simulink model "differential_drive_base_robot_current_loop"  (R2015b)
settings: Solver=VariableStepAuto  StartTime=0.0  StopTime=10.0  RelTol=1e-3
values from neighbouring files (symbols this model uses):
  B = 0.1    [andbot1dot2_modeling_param.m]    (also in andbot1dot2_param.m)
  J = 0.1    [andbot1dot2_modeling_param.m]    (also in andbot1dot2_param.m)
  m = 18.8    [andbot1dot2_modeling_param.m]    (also in andbot1dot2_param.m)
  r = 0.085    [andbot1dot2_modeling_param.m]    (also in andbot1dot2_param.m)
undefined symbols (not defined in the file or in its folder): km
settings Model: Creator=shangwei  LastModifiedBy=shangwei

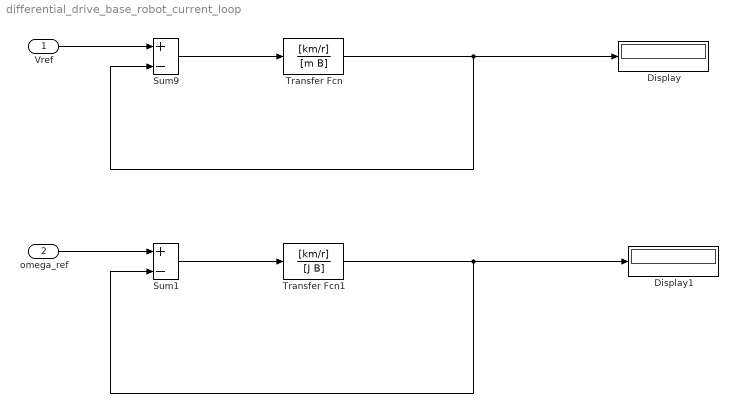
== system differential_drive_base_robot_current_loop ==
  Vref : Inport
  omega_ref : Inport  Port=2
  Display : Display
  Display1 : Display
  Sum1 : Sum  Inputs=+-
  Sum9 : Sum  Inputs=+-
  Transfer Fcn : TransferFcn  Numerator=[km/r]  Denominator=[m B]
  Transfer Fcn1 : TransferFcn  Numerator=[km/r]  Denominator=[J B]
  wires:
  Sum9/1 -> Transfer Fcn/1
  Transfer Fcn/1 -> Sum9/2, Display/1
  Vref/1 -> Sum9/1
  Sum1/1 -> Transfer Fcn1/1
  omega_ref/1 -> Sum1/1
  Transfer Fcn1/1 -> Sum1/2, Display1/1
